simulink model "pend_lib"  (Simulink 7.1)
settings: Solver=ode45  StartTime=0.0  StopTime=10.0  RelTol=1e-3
values from neighbouring files (symbols this model uses):
  g = 9.81    [MPCsimulink.m]    (also in assignment4.m; pend_init.m; setupOptimization.m)
  g1 = c2d(tf([1 0],[tcAngleVel 1]),h,'tustin')    [assignment4.m]    (also in assignment5.m; pend_init.m)
  g2 = c2d(tf(1,[tcAngle 1]),h,'tustin')    [assignment4.m]    (also in assignment5.m; pend_init.m)
  g3 = c2d(tf(1),h)    [assignment1.m]    (also in assignment3.m = c2d(tf(1,[tcAcc 1]),h,'tustin'); assignment4.m = c2d(tf(1,[tcAcc 1]),h,'tustin'); assignment5.m = c2d(tf(1,[tcAcc 1]),h,'tustin'); pend_init.m = c2d(tf(1,[tcAcc 1]),h,'tustin'))
  h = uIn(5*N+10)    [MPCsimulink.m]    (also in assignment1.m = 0.001; pend_init.m = 0.01)
  initPendValue = [0;0]    [assignment3.m]    (also in assignment4.m; pend_init.m)
  initPosError = 0    [assignment1.m]    (also in assignment3.m; assignment4.m; assignment5.m; pend_init.m)
  l = 0.345    [MPCsimulink.m]    (also in assignment4.m; loaddym.m = fgetl(fid); pend_init.m)
  p0 = -1.5    [assignment1.m]    (also in assignment5.m = -0.8)
undefined symbols (not defined in the file or in its folder): DiscIntNeverNeededParam
libraries: simulink x1
settings Model: Creator=pontusg  LastModifiedBy=pontusg  ExtModeAutoUpdateStatusClock=off
settings DebuggingCC: SaveWithParameterizedLinksMsg=none
settings GRTTargetCC: TargetFcnLib=ansi_tfl_tmw.mat

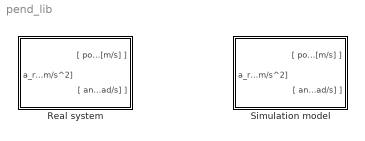
== system pend_lib ==
  Real system : Subsystem
  Simulation model : Subsystem

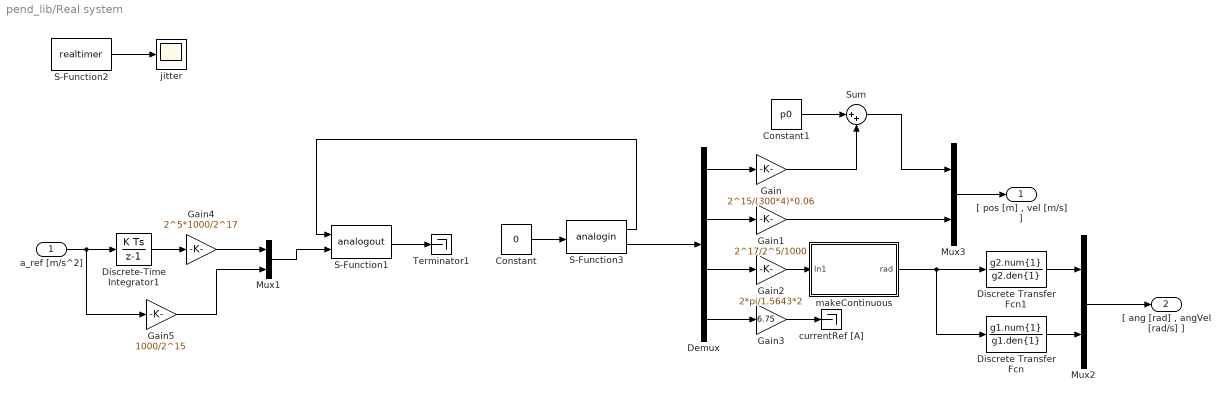
== system pend_lib/Real system ==
  a_ref [m/s^2] : Inport  OutDataType=sfix(16)  OutScaling=2^0
  Constant : Constant  Value=0  OutDataType=sfix(16)  OutScaling=2^0
  Constant1 : Constant  Value=p0  OutDataType=sfix(16)  OutScaling=2^0
  Demux : Demux
  Discrete Transfer Fcn : DiscreteTransferFcn  Numerator=g1.num{1}  Denominator=g1.den{1}  SampleTime=h
  Discrete Transfer Fcn1 : DiscreteTransferFcn  Numerator=g2.num{1}  Denominator=g2.den{1}  SampleTime=h
  Discrete-Time Integrator1 : DiscreteIntegrator  SampleTime=h  OutDataType=sfix(16)  OutScaling=2^0  ICPrevOutput=DiscIntNeverNeededParam  ICPrevScaledInput=DiscIntNeverNeededParam
  Gain : Gain  Gain=2^15/(300*4)*0.06  ParameterDataType=sfix(16)  ParameterScaling=2^0  OutDataType=sfix(16)  OutScaling=2^0
  Gain1 : Gain  Gain=2^17/2^5/1000  ParameterDataType=sfix(16)  ParameterScaling=2^0  OutDataType=sfix(16)  OutScaling=2^0
  Gain2 : Gain  Gain=2*pi/1.5643*2  ParameterDataType=sfix(16)  ParameterScaling=2^0  OutDataType=sfix(16)  OutScaling=2^0
  Gain3 : Gain  Gain=6.75  ParameterDataType=sfix(16)  ParameterScaling=2^0  OutDataType=sfix(16)  OutScaling=2^0
  Gain4 : Gain  Gain=2^5*1000/2^17  ParameterDataType=sfix(16)  ParameterScaling=2^0  OutDataType=sfix(16)  OutScaling=2^0
  Gain5 : Gain  Gain=1000/2^15  ParameterDataType=sfix(16)  ParameterScaling=2^0  OutDataType=sfix(16)  OutScaling=2^0
  Mux1 : Mux  Inputs=2
  Mux2 : Mux  Inputs=2
  Mux3 : Mux  Inputs=2
  S-Function1 : S-Function  FunctionName=analogout  Parameters=h [30 31]  EnableBusSupport=off
  S-Function2 : S-Function  FunctionName=realtimer  Parameters=h  EnableBusSupport=off
  S-Function3 : S-Function  FunctionName=analogin  Parameters=h [30 31 32 33]  EnableBusSupport=off
  Sum : Sum  Inputs=|++  OutDataType=sfix(16)  OutScaling=2^0
  Terminator1 : Terminator
  currentRef [A] : Terminator
  jitter : Scope
      settings: TickLabels=on  YMin=1  YMax=1  DataFormat=Array
  makeContinuous : Subsystem
  "[ pos [m] , vel [m/s] ]" : Outport  OutDataType=sfix(16)  OutScaling=2^0
  "[ ang [rad] , angVel [rad/s] ]" : Outport  Port=2  OutDataType=sfix(16)  OutScaling=2^0
  wires:
  S-Function2/1 -> jitter/1
  a_ref [m/s^2]/1 -> Gain5/1, Discrete-Time Integrator1/1
  Constant/1 -> S-Function3/1
  S-Function3/1 -> S-Function1/1
  S-Function3/2 -> Demux/1
  Demux/1 -> Gain/1
  Demux/2 -> Gain1/1
  Gain1/1 -> Mux3/2
  Demux/3 -> Gain2/1
  Demux/4 -> Gain3/1
  Gain2/1 -> makeContinuous/1(In1)
  Discrete-Time Integrator1/1 -> Gain4/1
  S-Function1/1 -> Terminator1/1
  Gain4/1 -> Mux1/1
  Gain5/1 -> Mux1/2
  Mux1/1 -> S-Function1/2
  Gain3/1 -> currentRef [A]/1
  makeContinuous/1(rad) -> Discrete Transfer Fcn1/1, Discrete Transfer Fcn/1
  Discrete Transfer Fcn1/1 -> Mux2/1
  Discrete Transfer Fcn/1 -> Mux2/2
  Mux2/1 -> "[ ang [rad] , angVel [rad/s] ]"/1
  Mux3/1 -> "[ pos [m] , vel [m/s] ]"/1
  Gain/1 -> Sum/2
  Constant1/1 -> Sum/1
  Sum/1 -> Mux3/1

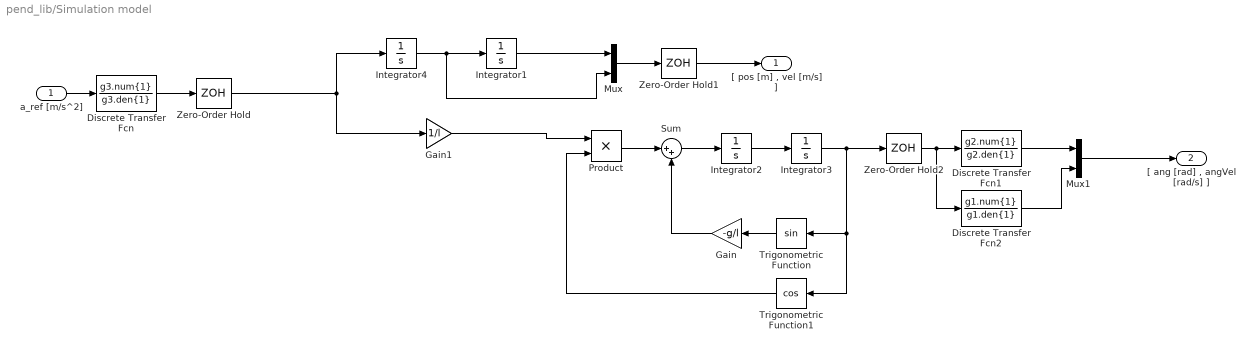
== system pend_lib/Simulation model ==
  a_ref [m/s^2] : Inport  OutDataType=sfix(16)  OutScaling=2^0
  Discrete Transfer Fcn : DiscreteTransferFcn  Numerator=g3.num{1}  Denominator=g3.den{1}  SampleTime=h
  Discrete Transfer Fcn1 : DiscreteTransferFcn  Numerator=g2.num{1}  Denominator=g2.den{1}  SampleTime=h
  Discrete Transfer Fcn2 : DiscreteTransferFcn  Numerator=g1.num{1}  Denominator=g1.den{1}  SampleTime=h
  Gain : Gain  Orientation=left  Gain=-g/l  ParameterDataType=sfix(16)  ParameterScaling=2^0  OutDataType=sfix(16)  OutScaling=2^0
  Gain1 : Gain  Gain=1/l  ParameterDataType=sfix(16)  ParameterScaling=2^0  OutDataType=sfix(16)  OutScaling=2^0
  Integrator1 : Integrator  InitialCondition=p0+initPosError
  Integrator2 : Integrator  InitialCondition=initPendValue(2)
  Integrator3 : Integrator  InitialCondition=initPendValue(1)
  Integrator4 : Integrator
  Mux : Mux  Inputs=2
  Mux1 : Mux  Inputs=2
  Product : Product  OutDataType=sfix(16)  OutScaling=2^0  RndMeth=Zero
  Sum : Sum  Inputs=|++  OutDataType=sfix(16)  OutScaling=2^0
  Trigonometric Function : Trigonometry  Orientation=left
  Trigonometric Function1 : Trigonometry  Orientation=left  Operator=cos
  Zero-Order Hold : ZeroOrderHold  SampleTime=h
  Zero-Order Hold1 : ZeroOrderHold  SampleTime=h
  Zero-Order Hold2 : ZeroOrderHold  SampleTime=h
  "[ pos [m] , vel [m/s] ]" : Outport  OutDataType=sfix(16)  OutScaling=2^0
  "[ ang [rad] , angVel [rad/s] ]" : Outport  Port=2  OutDataType=sfix(16)  OutScaling=2^0
  wires:
  Zero-Order Hold1/1 -> "[ pos [m] , vel [m/s] ]"/1
  Zero-Order Hold/1 -> Gain1/1, Integrator4/1
  Integrator4/1 -> Integrator1/1, Mux/2
  Integrator1/1 -> Mux/1
  Integrator2/1 -> Integrator3/1
  Integrator3/1 -> Trigonometric Function/1, Trigonometric Function1/1, Zero-Order Hold2/1
  Sum/1 -> Integrator2/1
  Mux/1 -> Zero-Order Hold1/1
  Mux1/1 -> "[ ang [rad] , angVel [rad/s] ]"/1
  a_ref [m/s^2]/1 -> Discrete Transfer Fcn/1
  Gain1/1 -> Product/1
  Product/1 -> Sum/1
  Trigonometric Function1/1 -> Product/2
  Trigonometric Function/1 -> Gain/1
  Gain/1 -> Sum/2
  Discrete Transfer Fcn1/1 -> Mux1/1
  Discrete Transfer Fcn2/1 -> Mux1/2
  Zero-Order Hold2/1 -> Discrete Transfer Fcn1/1, Discrete Transfer Fcn2/1
  Discrete Transfer Fcn/1 -> Zero-Order Hold/1

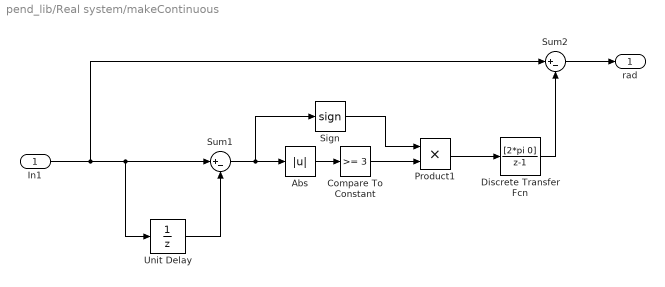
== system pend_lib/Real system/makeContinuous ==
  In1 : Inport  OutDataType=sfix(16)  OutScaling=2^0
  Abs : Abs
  Compare To Constant : simulink/Logic and Bit Operations/Compare To Constant  SystemSampleTime=-1  relop=>=  const=3  LogicOutDataTypeMode=uint8  ZeroCross=off
  Discrete Transfer Fcn : DiscreteTransferFcn  Numerator=[2*pi 0]  Denominator=[1 -1]  SampleTime=-1
  Product1 : Product  OutDataType=sfix(16)  OutScaling=2^0  RndMeth=Zero
  Sign : Signum
  Sum1 : Sum  Inputs=|+-  OutDataType=sfix(16)  OutScaling=2^0
  Sum2 : Sum  Inputs=|+-  OutDataType=sfix(16)  OutScaling=2^0
  Unit Delay : UnitDelay  SampleTime=-1
  rad : Outport  OutDataType=sfix(16)  OutScaling=2^0
  wires:
  Discrete Transfer Fcn/1 -> Sum2/2
  Product1/1 -> Discrete Transfer Fcn/1
  Sign/1 -> Product1/1
  Compare To Constant/1 -> Product1/2
  Sum2/1 -> rad/1
  Abs/1 -> Compare To Constant/1
  Sum1/1 -> Sign/1, Abs/1
  Unit Delay/1 -> Sum1/2
  In1/1 -> Sum2/1, Sum1/1, Unit Delay/1
